simulink model "slrt_filelog_minimal"  (R2023b)
settings: Solver=FixedStepDiscrete  StartTime=0.0  StopTime=5  FixedStep=0.001  RelTol=1e-3
libraries: slrealtimeloglib x3
settings Model: Creator=Administrator  LastModifiedBy=Administrator
settings SolverCC: ConcurrentTasks=on  PositivePriorityOrder=on
settings OptimizationCC: BlockReduction=off  OptimizeBlockIOStorage=off
settings DebuggingCC: TasksWithSamePriorityMsg=none
settings HardwareCC: ProdBitPerLong=64  ProdLongLongMode=on  ProdHWDeviceType=Intel->x86-64 (Linux 64)
settings RTWCC: Description=Simulink Real-Time  SystemTargetFile=slrealtime.tlc  TemplateMakefile=slrealtime_default_tmf  RTWVerbose=off  Toolchain=Simulink Real-Time Toolchain  BuildConfiguration=Faster Runs  CodeExecutionProfiling=on  TargetLang=C++
settings SimulinkRealTimeTargetCC: SLRTFileLogMaxRuns=10

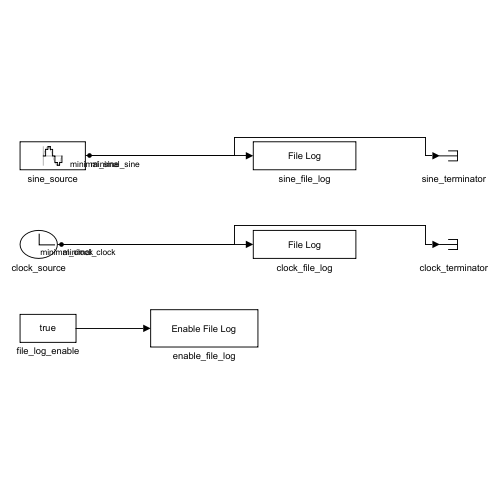
[thumbnail: Simulink's stored preview of the top-level diagram]
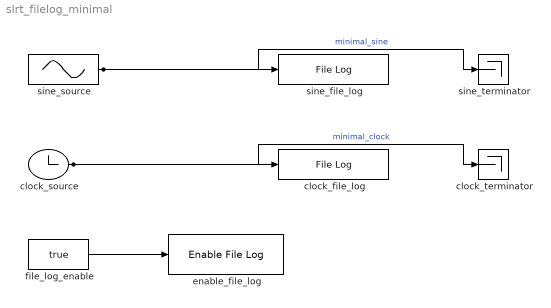
== system slrt_filelog_minimal ==
  clock_file_log : slrealtimeloglib/File Log  decimation=1  inputProcessing=Elements as channels (sample based)
  clock_source : Clock
  clock_terminator : Terminator
  enable_file_log : slrealtimeloglib/Enable File Log
  file_log_enable : Constant  Value=true  OutDataTypeStr=boolean
  sine_file_log : slrealtimeloglib/File Log  decimation=1  inputProcessing=Elements as channels (sample based)
  sine_source : Sin  Frequency=2*pi*1  SampleTime=0.001
  sine_terminator : Terminator
  wires:
  sine_source/1 -> sine_file_log/1, sine_terminator/1  "minimal_sine"
  clock_source/1 -> clock_file_log/1, clock_terminator/1  "minimal_clock"
  file_log_enable/1 -> enable_file_log/1
